simulink library "uavsimBlockset_Quaternion2Rotationvector"  (Simulink 8.0)
settings: Solver=ode45  StartTime=0.0  StopTime=10.0  RelTol=1e-3
libraries: uavsimBlockset_UnitVector x1
settings Model: Creator=mstolle  LastModifiedBy=j.bolting

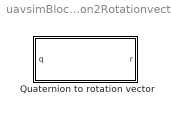
== system uavsimBlockset_Quaternion2Rotationvector ==
  Quaternion to rotation vector : Subsystem

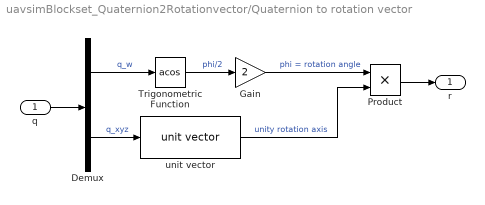
== system uavsimBlockset_Quaternion2Rotationvector/Quaternion to rotation vector ==
  q : Inport
  Demux : Demux  Outputs=[1 3]
  Gain : Gain  Gain=2
  Product : Product  RndMeth=Zero
  Trigonometric Function : Trigonometry  Operator=acos
  unit vector : uavsimBlockset_UnitVector/unit vector
  r : Outport
  wires:
  Trigonometric Function/1 -> Gain/1  "phi/2"
  q/1 -> Demux/1
  Demux/1 -> Trigonometric Function/1  "q_w"
  Demux/2 -> unit vector/1  "q_xyz"
  Gain/1 -> Product/1  "phi = rotation angle"
  unit vector/1 -> Product/2  "unity rotation axis"
  Product/1 -> r/1
